simulink model "testSubsystem"  (Simulink 7.4)
settings: Solver=ode45  StartTime=0.0  StopTime=10.0  RelTol=1e-3
libraries: BLOM_Lib x2
settings Model: Creator=Eric  LastModifiedBy=Eric

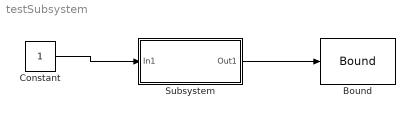
== system testSubsystem ==
  Bound : BLOM_Lib/Bound  SystemSampleTime=-1  ub=1  lb=0  initial_step=on  final_step=on  intermediate_step=on
  Constant : Constant  OutDataType=fixdt(1, 16)  OutScaling=2^0
  Subsystem : Subsystem
  wires:
  Constant/1 -> Subsystem/1(In1)
  Subsystem/1(Out1) -> Bound/1

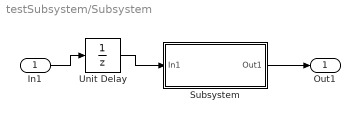
== system testSubsystem/Subsystem ==
  In1 : Inport  OutDataType=fixdt(1, 16)  OutScaling=2^0
  Subsystem : Subsystem
  Unit Delay : UnitDelay  SampleTime=-1
  Out1 : Outport  OutDataType=fixdt(1, 16)  OutScaling=2^0
  wires:
  In1/1 -> Unit Delay/1
  Subsystem/1(Out1) -> Out1/1
  Unit Delay/1 -> Subsystem/1(In1)

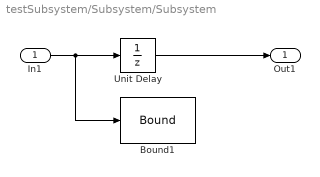
== system testSubsystem/Subsystem/Subsystem ==
  In1 : Inport  OutDataType=fixdt(1, 16)  OutScaling=2^0
  Bound1 : BLOM_Lib/Bound  SystemSampleTime=-1  ub=2  lb=1  initial_step=on  final_step=on  intermediate_step=on
  Unit Delay : UnitDelay  SampleTime=-1
  Out1 : Outport  OutDataType=fixdt(1, 16)  OutScaling=2^0
  wires:
  In1/1 -> Unit Delay/1, Bound1/1
  Unit Delay/1 -> Out1/1
